simulink model "msj"  (R2018b)
settings: Solver=VariableStepAuto  StartTime=0.0  StopTime=8  RelTol=1e-3
undefined symbols (not defined in the file or in its folder): drawMSJ, force, P
settings Model: Creator=Yufeng Sun  LastModifiedBy=Yufeng Sun

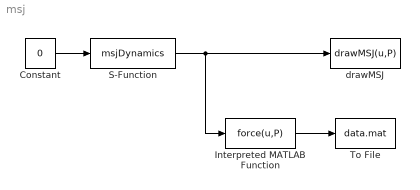
== system msj ==
  Constant : Constant  Value=0
  Interpreted MATLAB Function : MATLABFcn  MATLABFcn=force(u,P)  OutputDimensions=3
  S-Function : S-Function  FunctionName=msjDynamics  Parameters=P  SFunctionDeploymentMode=off  EnableBusSupport=off
  To File : ToFile  Filename=data.mat  SaveFormat=Timeseries
  drawMSJ : MATLABFcn  MATLABFcn=drawMSJ(u,P)  OutputDimensions=0
  wires:
  S-Function/1 -> Interpreted MATLAB Function/1, drawMSJ/1
  Constant/1 -> S-Function/1
  Interpreted MATLAB Function/1 -> To File/1
